simulink model "HVModAL_Fahrzeugmodell"  (R2015b)
settings: Solver=ode1  StartTime=0  StopTime=drp.driving_cycle.tstop  FixedStep=sim_params.Ts  RelTol=1e-5
PreLoadFcn:
  | % Add paths
  | addpath data
  | addpath(genpath('library'))
StartFcn:
  | Simulation.StartTime = tic;
StopFcn:
  | Simulation.DurationTime = toc(Simulation.StartTime);
undefined symbols (not defined in the file or in its folder): Batteries, BMS, BMS_Bat_, C_Nenn_DCDC1, C_Nenn_DCDC2, d2d, DC, DCDC_Converter_efficiency, DcDc_Converters, Dcl, drp, drv, elm, gen, gin, Hdc, hdc, HV, hvb, Hvb, ice, ldc, lib_dcl, lib_hdc, lib_hvb, lib_veh, Link, lossestable, mask_LUT_OCV, mask_LUT_OCV_SOC, mask_LUT_OCV_Temperature, mask_LUT_R, mask_LUT_Rs, mask_LUT_Rs_SOC, mask_LUT_Rs_Temperature, sim_params, speedvec, torquevec, tri, veh, Veh, Vehicle_Chassis
libraries: simulink x29, lib_tri_modules x7, lib_hdc_module x5, lib_gearbox x4, lib_hvb_battery_pack x3, cstblocks x3, PowerLimitBlock x2, MultiCellLibrary x2, lib_aux x1, lib_drv x1, lib_gen x1, lib_elm x1
(part 5 of 7)

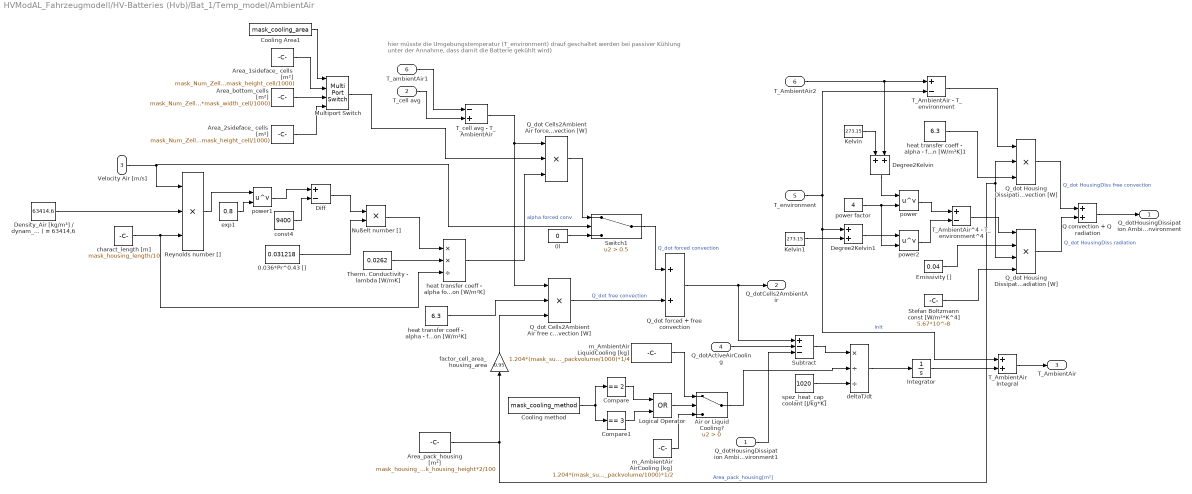
== system HVModAL_Fahrzeugmodell/HV-Batteries (Hvb)/Bat_1/Temp_model/AmbientAir ==
  note: hier müsste die Umgebungstemperatur (T_environment) drauf geschaltet werden bei passiver Kühlung
      | unter der Annahme, dass damit die Batterie gekühlt wird)
  Q_dotHousingDissipation AmbientAir2Environment1 : Inport
  T_cell avg : Inport  Port=2
  Velocity Air [m/s] : Inport  Port=3
  Q_dotActiveAirCooling : Inport  Port=4
  T_environment : Inport  Port=5
  T_AmbientAir2 : Inport  Port=6
  0.036*Pr^0.43 [] : Constant  Value=0.031218
  0l : Constant  Value=0
  Air or Liquid Cooling? : Switch  Criteria=u2 > Threshold
  Area_1sideface_ cells [m²] : Constant  Value=mask_Num_Zellen_el_ser*mask_Num_Zellen_el_par*(mask_width_cell/1000*mask_height_cell/1000)
  Area_2sideface_ cells [m²] : Constant  Value=mask_Num_Zellen_el_ser*mask_Num_Zellen_el_par*(2*mask_width_cell/1000*mask_height_cell/1000)
  Area_bottom_cells [m²] : Constant  Value=mask_Num_Zellen_el_ser*mask_Num_Zellen_el_par*(mask_thickness_cell/1000*mask_width_cell/1000)
  Area_pack_housing [m²] : Constant  Value=mask_housing_width*mask_housing_length*2/100+mask_housing_height*mask_housing_length*2/100+mask_housing_width*mask_housing_height*2/100
  Compare : simulink/Logic and Bit Operations/Compare To Constant  relop===  const=2  OutDataTypeStr=boolean
  Compare1 : simulink/Logic and Bit Operations/Compare To Constant  relop===  const=3  OutDataTypeStr=boolean
  Cooling Area1 : Constant  Value=mask_cooling_area
  Cooling method : Constant  Value=mask_cooling_method
  Degree2Kelvin : Sum
  Degree2Kelvin1 : Sum
  Density_Air [kg/m³] / dynam_visc_air @ 25°C [Pa*s] = 1,17 / (1,845*10^-5 ) = 63414,6 : Constant  Value=63414.6
  Diff : Sum  Inputs=+-
  Emissivity [] : Constant  Value=0.04
  Integrator : Integrator
  Kelvin : Constant  Value=273.15
  Kelvin1 : Constant  Value=273.15
  Logical Operator : Logic  Operator=OR  AllPortsSameDT=off  OutDataTypeStr=boolean
  Multiport Switch : MultiPortSwitch
  Nußelt number [] : Product
  Q convection + Q radiation : Sum
  Q_dot Cells2AmbientAir forced convection [W] : Product  Inputs=3
  Q_dot Cells2AmbientAir free convection [W] : Product  Inputs=3
  Q_dot Housing Dissipation free convection [W] : Product  Inputs=3
  Q_dot Housing Dissipation radiation [W] : Product  Inputs=4
  Q_dot forced + free convection : Sum
  Reynolds number [] : Product  Inputs=***
  Stefan Boltzmann const [W/m²*K^4] : Constant  Value=5.67*10^-8
  Subtract : Sum  Inputs=+--
  Switch1 : Switch  Criteria=u2 > Threshold  Threshold=0.5
  "T_AmbientAir Integral " : Sum
  T_AmbientAir - T_environment : Sum  Inputs=+-
  T_AmbientAir^4 - T_environment^4 : Sum  Inputs=+-
  T_ambientAir1 : InportShadow  Port=6
  T_cell avg - T_AmbientAir : Sum  Inputs=-+
  "Therm. Conductivity - lambda [W/mK] " : Constant  Value=0.0262
  charact_length [m] : Constant  Value=mask_housing_length/10
  const4 : Constant  Value=9400
  deltaT/dt : Product  Inputs=*//
  exp1 : Constant  Value=0.8
  factor_cell_area_housing_area : Gain  Gain=0.95
  heat transfer coeff - alpha forced convection [W/m²K] : Product  Inputs=**/
  heat transfer coeff - alpha - free convection [W/m²K] : Constant  Value=6.3
  heat transfer coeff - alpha - free convection [W/m²K]1 : Constant  Value=6.3
  m_AmbientAir AirCooling [kg] : Constant  Value=1.204*(mask_sum_packvolume/1000)*1/2
  m_AmbientAir LiquidCooling [kg] : Constant  Value=1.204*(mask_sum_packvolume/1000)*1/4
  power : Math  Operator=pow  SaturateOnIntegerOverflow=on
  power factor : Constant  Value=4
  power1 : Math  Operator=pow  SaturateOnIntegerOverflow=on
  power2 : Math  Operator=pow  SaturateOnIntegerOverflow=on
  spez_heat_cap_coolant [J/kg*K] : Constant  Value=1020
  Q_dotHousingDissipation AmbientAir2Environment : Outport
  Q_dotCells2AmbientAir : Outport  Port=2
  T_AmbientAir : Outport  Port=3
  wires:
  T_cell avg - T_AmbientAir/1 -> Q_dot Cells2AmbientAir free convection [W]/1, Q_dot Cells2AmbientAir forced convection [W]/1
  Q_dot forced + free convection/1 -> Q_dotCells2AmbientAir/1, Subtract/1
  T_cell avg/1 -> T_cell avg - T_AmbientAir/2
  Density_Air [kg/m³] / dynam_visc_air @ 25°C [Pa*s] = 1,17 / (1,845*10^-5 ) = 63414,6/1 -> Reynolds number []/2
  Reynolds number []/1 -> power1/1
  exp1/1 -> power1/2
  power1/1 -> Diff/1
  const4/1 -> Diff/2
  Diff/1 -> Nußelt number []/1
  "Therm. Conductivity - lambda [W/mK] "/1 -> heat transfer coeff - alpha forced convection [W/m²K]/2
  heat transfer coeff - alpha forced convection [W/m²K]/1 -> Q_dot Cells2AmbientAir forced convection [W]/3  "alpha forced conv"
  charact_length [m]/1 -> heat transfer coeff - alpha forced convection [W/m²K]/3, Reynolds number []/3
  Nußelt number []/1 -> heat transfer coeff - alpha forced convection [W/m²K]/1
  0.036*Pr^0.43 []/1 -> Nußelt number []/2
  Velocity Air [m/s]/1 -> Reynolds number []/1, Switch1/2
  0l/1 -> Switch1/3
  Q_dot Cells2AmbientAir forced convection [W]/1 -> Switch1/1
  Switch1/1 -> Q_dot forced + free convection/1  "Q_dot forced convection"
  Q_dot Cells2AmbientAir free convection [W]/1 -> Q_dot forced + free convection/2  "Q_dot free convection"
  heat transfer coeff - alpha - free convection [W/m²K]/1 -> Q_dot Cells2AmbientAir free convection [W]/2
  Multiport Switch/1 -> Q_dot Cells2AmbientAir forced convection [W]/2
  "T_AmbientAir Integral "/1 -> T_AmbientAir/1
  Subtract/1 -> deltaT/dt/1
  spez_heat_cap_coolant [J/kg*K]/1 -> deltaT/dt/3
  deltaT/dt/1 -> Integrator/1
  Integrator/1 -> "T_AmbientAir Integral "/2
  T_environment/1 -> T_AmbientAir - T_environment/2, Degree2Kelvin1/1, "T_AmbientAir Integral "/1  "init"
  T_AmbientAir - T_environment/1 -> Q_dot Housing Dissipation free convection [W]/1
  heat transfer coeff - alpha - free convection [W/m²K]1/1 -> Q_dot Housing Dissipation free convection [W]/3
  Area_pack_housing [m²]/1 -> Q_dot Housing Dissipation radiation [W]/3, Q_dot Housing Dissipation free convection [W]/2, factor_cell_area_housing_area/1  "Area_pack_housing[m²]"
  Q_dot Housing Dissipation free convection [W]/1 -> Q convection + Q radiation/1  "Q_dot HousingDIss free convection"
  Emissivity []/1 -> Q_dot Housing Dissipation radiation [W]/2
  Stefan Boltzmann const [W/m²*K^4]/1 -> Q_dot Housing Dissipation radiation [W]/4
  Q_dot Housing Dissipation radiation [W]/1 -> Q convection + Q radiation/2  "Q_dot HousingDiss radiation"
  Cooling method/1 -> Compare/1, Compare1/1
  Compare/1 -> Logical Operator/1
  Compare1/1 -> Logical Operator/2
  Logical Operator/1 -> Air or Liquid Cooling?/2
  Q_dotHousingDissipation AmbientAir2Environment1/1 -> Subtract/3
  power factor/1 -> power2/2, power/2
  Degree2Kelvin/1 -> power/1
  Kelvin/1 -> Degree2Kelvin/1
  T_ambientAir1/1 -> T_cell avg - T_AmbientAir/1
  T_AmbientAir2/1 -> T_AmbientAir - T_environment/1, Degree2Kelvin/2
  Q convection + Q radiation/1 -> Q_dotHousingDissipation AmbientAir2Environment/1
  Air or Liquid Cooling?/1 -> deltaT/dt/2
  m_AmbientAir AirCooling [kg]/1 -> Air or Liquid Cooling?/3
  T_AmbientAir^4 - T_environment^4/1 -> Q_dot Housing Dissipation radiation [W]/1
  power/1 -> T_AmbientAir^4 - T_environment^4/1
  Kelvin1/1 -> Degree2Kelvin1/2
  Degree2Kelvin1/1 -> power2/1
  power2/1 -> T_AmbientAir^4 - T_environment^4/2
  Q_dotActiveAirCooling/1 -> Subtract/2
  m_AmbientAir LiquidCooling [kg]/1 -> Air or Liquid Cooling?/1
  Area_bottom_cells [m²]/1 -> Multiport Switch/3
  Cooling Area1/1 -> Multiport Switch/1
  Area_1sideface_ cells [m²]/1 -> Multiport Switch/2
  Area_2sideface_ cells [m²]/1 -> Multiport Switch/4
  factor_cell_area_housing_area/1 -> Q_dot Cells2AmbientAir free convection [W]/3

== system HVModAL_Fahrzeugmodell/HV-Batteries (Hvb)/Bat_1/Temp_model/Cell ==
  Q_dot Cell2CoolingSystem+AmbientAir : Inport
  T_environment : Inport  Port=2
  Q_dot Loss Cell : Inport  Port=3
  C_Therm_Cell[J/K] : Constant  Value=1100*mask_m_cell
  Integrator : Integrator
  Q_dot Loss Cell - Q_dot Cell2CoolingSys+AmbAir : Sum  Inputs=+-
  T_cell avg Integral : Sum
  delta_T/dt : Product  Inputs=*/
  T_cell avg : Outport
  wires:
  C_Therm_Cell[J/K]/1 -> delta_T/dt/2
  delta_T/dt/1 -> Integrator/1
  Integrator/1 -> T_cell avg Integral/1
  Q_dot Loss Cell - Q_dot Cell2CoolingSys+AmbAir/1 -> delta_T/dt/1
  Q_dot Loss Cell/1 -> Q_dot Loss Cell - Q_dot Cell2CoolingSys+AmbAir/1
  T_cell avg Integral/1 -> T_cell avg/1
  Q_dot Cell2CoolingSystem+AmbientAir/1 -> Q_dot Loss Cell - Q_dot Cell2CoolingSys+AmbAir/2
  T_environment/1 -> T_cell avg Integral/2  "init"

== system HVModAL_Fahrzeugmodell/HV-Batteries (Hvb)/Bat_1/Temp_model/CoolingChannel ==
  note: 1 Elektrode Kupfer eine Alu,
      | d.h. unterschiedl. Lambdas?!
  T_environment : Inport
  T_cell avg [K] : Inport  Port=2
  Q_dot LiquidCoolingSystem : Inport  Port=3
  Q_dot PTC Heater : Inport  Port=4
  1/Thickness [1/m] : Constant  Value=1/0.006
  1/Thickness_Alu [1/m] : Constant  Value=1/0.007
  Area_1sideface_ cells [m²] : Constant  Value=mask_Num_Zellen_el_ser*mask_Num_Zellen_el_par*(mask_width_cell/1000*mask_height_cell/1000)
  Area_2sideface_ cells [m²] : Constant  Value=mask_Num_Zellen_el_ser*mask_Num_Zellen_el_par*(2*mask_width_cell/1000*mask_height_cell/1000)
  Area_bottom_cells [m²] : Constant  Value=mask_Num_Zellen_el_ser*mask_Num_Zellen_el_par*(mask_thickness_cell/1000*mask_width_cell/1000)
  Cooling Area : Constant  Value=mask_cooling_area
  Divide : Product  Inputs=*//
  Integrator : Integrator
  Multiport Switch : MultiPortSwitch
  T_ cell avg - T_Cooling Channel : Sum  Inputs=+-
  T_Cooling Channel Integral : Sum
  Temp-diff.2 : Sum  Inputs=+-
  Thermal Conductivity Alu - lambda [W/m*K] : Constant  Value=236
  Thermal Conductivity Alu - lambda [W/m*K] : Constant  Value=236
  delta_Q : Sum  Inputs=-++
  m_coolant [kg] : Constant  Value=7.28
  spez_heat_cap - c_p coolant : Constant  Value=2350
  therm conduction Cells2CoolingSystem : Product  Inputs=4
  therm_conduction Cells2Refrigerant : Product  Inputs=4
  Q_dot Cells2Refri : Outport
  Q_dot Cells2CoolingSystem : Outport  Port=2
  wires:
  Q_dot PTC Heater/1 -> delta_Q/3
  m_coolant [kg]/1 -> Divide/2
  spez_heat_cap - c_p coolant/1 -> Divide/3
  Divide/1 -> Integrator/1
  Integrator/1 -> T_Cooling Channel Integral/2
  delta_Q/1 -> Divide/1
  therm conduction Cells2CoolingSystem/1 -> Q_dot Cells2CoolingSystem/1, delta_Q/2
  1/Thickness [1/m]/1 -> therm conduction Cells2CoolingSystem/4
  T_ cell avg - T_Cooling Channel/1 -> therm conduction Cells2CoolingSystem/3
  T_Cooling Channel Integral/1 -> Temp-diff.2/1, T_ cell avg - T_Cooling Channel/2
  Thermal Conductivity Alu - lambda [W/m*K]/1 -> therm conduction Cells2CoolingSystem/2
  Q_dot LiquidCoolingSystem/1 -> delta_Q/1
  Thermal Conductivity Alu - lambda [W/m*K]/1 -> therm_conduction Cells2Refrigerant/2
  1/Thickness_Alu [1/m]/1 -> therm_conduction Cells2Refrigerant/4
  Multiport Switch/1 -> therm_conduction Cells2Refrigerant/1, therm conduction Cells2CoolingSystem/1
  Temp-diff.2/1 -> therm_conduction Cells2Refrigerant/3
  T_cell avg [K]/1 -> Temp-diff.2/2, T_ cell avg - T_Cooling Channel/1
  therm_conduction Cells2Refrigerant/1 -> Q_dot Cells2Refri/1
  T_environment/1 -> T_Cooling Channel Integral/1  "init"
  Area_bottom_cells [m²]/1 -> Multiport Switch/3
  Cooling Area/1 -> Multiport Switch/1
  Area_1sideface_ cells [m²]/1 -> Multiport Switch/2
  Area_2sideface_ cells [m²]/1 -> Multiport Switch/4

== system HVModAL_Fahrzeugmodell/HV-Batteries (Hvb)/Bat_1/Temp_model/LiquidCoolingCompressor ==
  note: 0: No cooling
      | 1: Active Aircooling
      | 2: Refrigerant Cooling
      | 3: Liquid Cooling
      | 4:Passive Aircooling
  Forced Cooled Coolant Cooling on : Inport
  Active Heating on : Inport  Port=2
  Compressor Power Factor : Inport  Port=3
  ComprCool off : Constant  Value=0
  LiquidCooling : Constant  Value=3
  Logical Op2 : Logic  AllPortsSameDT=off  OutDataTypeStr=boolean
  Null2 : Constant  Value=0
  P_max PTC Heater : Constant  Value=mask_P_max_disch*0.02
  P_max LiquidCoolingSys : Constant  Value=mask_P_max_disch*0.02
  P_max_compr [W] : Gain  Gain=mask_P_max_disch*0.02
  P_max_compr [W]1 : Gain  Gain=mask_P_max_disch*0.02
  RellOp : RelationalOperator  Operator===  OutDataTypeStr=boolean
  Switch : Switch  Criteria=u2 > Threshold  Threshold=1
  Switch3 : Switch  Criteria=u2 ~= 0  Threshold=1
  Switch4 : Switch  Criteria=u2 ~= 0  Threshold=20
  Switch5 : Switch  Criteria=u2 > Threshold  Threshold=1
  cooling system : Constant  Value=mask_cooling_method
  Q_dot LiquidCoolingSystem : Outport
  Q_dot PTC Heater : Outport  Port=2
  wires:
  P_max_compr [W]/1 -> Switch/3
  Compressor Power Factor/1 -> Switch5/2, P_max_compr [W]1/1, Switch/2, P_max_compr [W]/1
  Switch/1 -> Switch3/1
  ComprCool off/1 -> Switch3/3
  Switch4/1 -> Q_dot PTC Heater/1
  Null2/1 -> Switch4/3
  P_max PTC Heater/1 -> Switch5/1
  P_max_compr [W]1/1 -> Switch5/3
  Switch5/1 -> Switch4/1
  Switch3/1 -> Q_dot LiquidCoolingSystem/1
  Active Heating on/1 -> Switch4/2
  P_max LiquidCoolingSys/1 -> Switch/1
  cooling system/1 -> RellOp/1
  LiquidCooling/1 -> RellOp/2
  Forced Cooled Coolant Cooling on/1 -> Logical Op2/1
  RellOp/1 -> Logical Op2/2
  Logical Op2/1 -> Switch3/2

== system HVModAL_Fahrzeugmodell/HV-Batteries (Hvb)/Bat_2/BMS_Bat_/Temp Regulation ==
  note: ActiveCoolingSwitchOnTemperature
  note: @ Mitsubishi i-MiEV:
      | Active AirCooling at fastcharging with battery temperature above 30°C
      | Passive AirCooling only at battery temperature above 25°C
  note: ActiveCoolingSwitchOffTemperature
  note: ActiveHeatingSwitchOnTemperature
  note: ActiveHeatingSwitchOffTemperature
  note: 0: No cooling
      | 1: Active Aircooling
      | 2: Refrigerant Cooling
      | 3: Liquid Cooling
      | 4:Passive Aircooling
  T_max : Inport
  Fast charging on : Inport  Port=2
  Abs : Abs
  Active AirCooling : Constant
  Compare : simulink/Logic and Bit Operations/Compare To Constant  relop=>=  const=30  OutDataTypeStr=boolean
  Compare1 : simulink/Logic and Bit Operations/Compare To Constant  relop=<  const=0  OutDataTypeStr=boolean
  Cooling on : Constant  Value=4
  Gain : Gain  Gain=1/20
  Liquid Cooling : Constant  Value=3
  Logical Op1 : Logic  Operator=OR  AllPortsSameDT=off  OutDataTypeStr=boolean
  Logical Op2 : Logic  Operator=OR  AllPortsSameDT=off  OutDataTypeStr=boolean
  Logical Operator : Logic  AllPortsSameDT=off  OutDataTypeStr=boolean
  Logical Op : Logic  AllPortsSameDT=off  OutDataTypeStr=boolean
  RelOp1 : RelationalOperator  Operator===  OutDataTypeStr=boolean
  RelOp2 : RelationalOperator  Operator===  OutDataTypeStr=boolean
  Relay : Relay  OnSwitchValue=25  OffSwitchValue=20
  RellOp : RelationalOperator  Operator===  OutDataTypeStr=boolean
  Sum : Sum  Inputs=|+-
  T_desired : Constant  Value=20
  Terminator1 : Terminator
  Velocity Air [m/s] : Constant  Value=mask_v_Radial_Fan
  cooling system : Constant  Value=mask_cooling_method
  Compressor Power Factor : Outport
  Forced Air Cooling on : Outport  Port=2
  Forced Cooled Coolant Cooling on : Outport  Port=3
  Active Heating on : Outport  Port=4
  Velocity Air : Outport  Port=5
  wires:
  T_desired/1 -> Sum/1
  T_max/1 -> Compare/1, Compare1/1, Relay/1, Sum/2
  Fast charging on/1 -> Logical Operator/2
  Compare/1 -> Logical Operator/1
  Logical Operator/1 -> Terminator1/1
  Sum/1 -> Abs/1
  Abs/1 -> Gain/1
  Gain/1 -> Compressor Power Factor/1
  Cooling on/1 -> RellOp/2
  cooling system/1 -> RelOp1/1, RelOp2/1, RellOp/1
  RellOp/1 -> Logical Op2/1
  Relay/1 -> Logical Op/2
  Active AirCooling/1 -> RelOp1/2
  Liquid Cooling/1 -> RelOp2/2
  Logical Op/1 -> Forced Cooled Coolant Cooling on/1
  Compare1/1 -> Active Heating on/1
  RelOp1/1 -> Logical Op2/2, Logical Op1/1
  Velocity Air [m/s]/1 -> Velocity Air/1
  Logical Op2/1 -> Forced Air Cooling on/1
  RelOp2/1 -> Logical Op1/2
  Logical Op1/1 -> Logical Op/1

== system HVModAL_Fahrzeugmodell/HV-Batteries (Hvb)/Bat_2/Temp_model/ActiveAirCoolingCompressor ==
  note: 0: No cooling
      | 1: Active Aircooling
      | 2: Refrigerant Cooling
      | 3: Liquid Cooling
      | 4:Passive Aircooling
  ForcedAir Cooling on : Inport
  Forced Cooled Coolant Cooling on : Inport  Port=2
  Compressor Power Factor : Inport  Port=3
  Velocity Airstream : Inport  Port=4
  Active AirCooling : Constant
  Logical Op2 : Logic  AllPortsSameDT=off  OutDataTypeStr=boolean
  No convection : Constant  Value=0
  P_max LiquidCoolingSys : Constant  Value=mask_P_max_disch*0.02
  P_max_compr [W] : Gain  Gain=mask_P_max_disch*0.02
  RellOp : RelationalOperator  Operator===  OutDataTypeStr=boolean
  Switch : Switch  Criteria=u2 > Threshold  Threshold=1
  Switch1 : Switch  Criteria=u2 ~= 0  Threshold=1
  Switch3 : Switch  Criteria=u2 ~= 0  Threshold=1
  air_con_compr off : Constant  Value=0
  cooling system : Constant  Value=mask_cooling_method
  Velocity Air : Outport
  Q_dotActiveAirCooling : Outport  Port=2
  wires:
  air_con_compr off/1 -> Switch1/3
  Velocity Airstream/1 -> Switch3/1
  No convection/1 -> Switch3/3
  Switch3/1 -> Velocity Air/1
  Switch1/1 -> Q_dotActiveAirCooling/1
  ForcedAir Cooling on/1 -> Switch3/2
  P_max_compr [W]/1 -> Switch/3
  Compressor Power Factor/1 -> Switch/2, P_max_compr [W]/1
  Switch/1 -> Switch1/1
  P_max LiquidCoolingSys/1 -> Switch/1
  Forced Cooled Coolant Cooling on/1 -> Logical Op2/1
  RellOp/1 -> Logical Op2/2
  cooling system/1 -> RellOp/1
  Active AirCooling/1 -> RellOp/2
  Logical Op2/1 -> Switch1/2

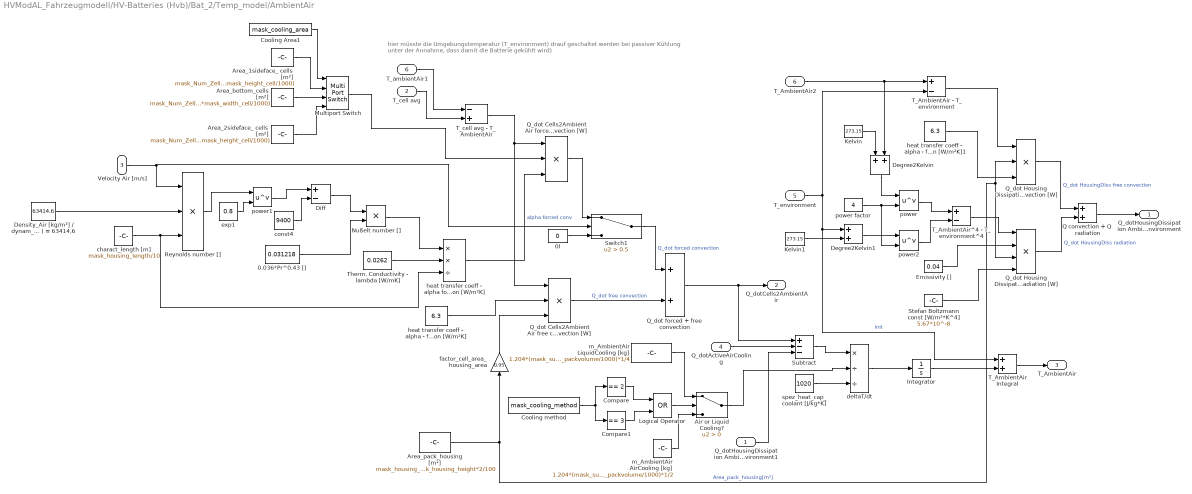
== system HVModAL_Fahrzeugmodell/HV-Batteries (Hvb)/Bat_2/Temp_model/AmbientAir ==
  note: hier müsste die Umgebungstemperatur (T_environment) drauf geschaltet werden bei passiver Kühlung
      | unter der Annahme, dass damit die Batterie gekühlt wird)
  Q_dotHousingDissipation AmbientAir2Environment1 : Inport
  T_cell avg : Inport  Port=2
  Velocity Air [m/s] : Inport  Port=3
  Q_dotActiveAirCooling : Inport  Port=4
  T_environment : Inport  Port=5
  T_AmbientAir2 : Inport  Port=6
  0.036*Pr^0.43 [] : Constant  Value=0.031218
  0l : Constant  Value=0
  Air or Liquid Cooling? : Switch  Criteria=u2 > Threshold
  Area_1sideface_ cells [m²] : Constant  Value=mask_Num_Zellen_el_ser*mask_Num_Zellen_el_par*(mask_width_cell/1000*mask_height_cell/1000)
  Area_2sideface_ cells [m²] : Constant  Value=mask_Num_Zellen_el_ser*mask_Num_Zellen_el_par*(2*mask_width_cell/1000*mask_height_cell/1000)
  Area_bottom_cells [m²] : Constant  Value=mask_Num_Zellen_el_ser*mask_Num_Zellen_el_par*(mask_thickness_cell/1000*mask_width_cell/1000)
  Area_pack_housing [m²] : Constant  Value=mask_housing_width*mask_housing_length*2/100+mask_housing_height*mask_housing_length*2/100+mask_housing_width*mask_housing_height*2/100
  Compare : simulink/Logic and Bit Operations/Compare To Constant  relop===  const=2  OutDataTypeStr=boolean
  Compare1 : simulink/Logic and Bit Operations/Compare To Constant  relop===  const=3  OutDataTypeStr=boolean
  Cooling Area1 : Constant  Value=mask_cooling_area
  Cooling method : Constant  Value=mask_cooling_method
  Degree2Kelvin : Sum
  Degree2Kelvin1 : Sum
  Density_Air [kg/m³] / dynam_visc_air @ 25°C [Pa*s] = 1,17 / (1,845*10^-5 ) = 63414,6 : Constant  Value=63414.6
  Diff : Sum  Inputs=+-
  Emissivity [] : Constant  Value=0.04
  Integrator : Integrator
  Kelvin : Constant  Value=273.15
  Kelvin1 : Constant  Value=273.15
  Logical Operator : Logic  Operator=OR  AllPortsSameDT=off  OutDataTypeStr=boolean
  Multiport Switch : MultiPortSwitch
  Nußelt number [] : Product
  Q convection + Q radiation : Sum
  Q_dot Cells2AmbientAir forced convection [W] : Product  Inputs=3
  Q_dot Cells2AmbientAir free convection [W] : Product  Inputs=3
  Q_dot Housing Dissipation free convection [W] : Product  Inputs=3
  Q_dot Housing Dissipation radiation [W] : Product  Inputs=4
  Q_dot forced + free convection : Sum
  Reynolds number [] : Product  Inputs=***
  Stefan Boltzmann const [W/m²*K^4] : Constant  Value=5.67*10^-8
  Subtract : Sum  Inputs=+--
  Switch1 : Switch  Criteria=u2 > Threshold  Threshold=0.5
  "T_AmbientAir Integral " : Sum
  T_AmbientAir - T_environment : Sum  Inputs=+-
  T_AmbientAir^4 - T_environment^4 : Sum  Inputs=+-
  T_ambientAir1 : InportShadow  Port=6
  T_cell avg - T_AmbientAir : Sum  Inputs=-+
  "Therm. Conductivity - lambda [W/mK] " : Constant  Value=0.0262
  charact_length [m] : Constant  Value=mask_housing_length/10
  const4 : Constant  Value=9400
  deltaT/dt : Product  Inputs=*//
  exp1 : Constant  Value=0.8
  factor_cell_area_housing_area : Gain  Gain=0.95
  heat transfer coeff - alpha forced convection [W/m²K] : Product  Inputs=**/
  heat transfer coeff - alpha - free convection [W/m²K] : Constant  Value=6.3
  heat transfer coeff - alpha - free convection [W/m²K]1 : Constant  Value=6.3
  m_AmbientAir AirCooling [kg] : Constant  Value=1.204*(mask_sum_packvolume/1000)*1/2
  m_AmbientAir LiquidCooling [kg] : Constant  Value=1.204*(mask_sum_packvolume/1000)*1/4
  power : Math  Operator=pow  SaturateOnIntegerOverflow=on
  power factor : Constant  Value=4
  power1 : Math  Operator=pow  SaturateOnIntegerOverflow=on
  power2 : Math  Operator=pow  SaturateOnIntegerOverflow=on
  spez_heat_cap_coolant [J/kg*K] : Constant  Value=1020
  Q_dotHousingDissipation AmbientAir2Environment : Outport
  Q_dotCells2AmbientAir : Outport  Port=2
  T_AmbientAir : Outport  Port=3
  wires:
  T_cell avg - T_AmbientAir/1 -> Q_dot Cells2AmbientAir free convection [W]/1, Q_dot Cells2AmbientAir forced convection [W]/1
  Q_dot forced + free convection/1 -> Q_dotCells2AmbientAir/1, Subtract/1
  T_cell avg/1 -> T_cell avg - T_AmbientAir/2
  Density_Air [kg/m³] / dynam_visc_air @ 25°C [Pa*s] = 1,17 / (1,845*10^-5 ) = 63414,6/1 -> Reynolds number []/2
  Reynolds number []/1 -> power1/1
  exp1/1 -> power1/2
  power1/1 -> Diff/1
  const4/1 -> Diff/2
  Diff/1 -> Nußelt number []/1
  "Therm. Conductivity - lambda [W/mK] "/1 -> heat transfer coeff - alpha forced convection [W/m²K]/2
  heat transfer coeff - alpha forced convection [W/m²K]/1 -> Q_dot Cells2AmbientAir forced convection [W]/3  "alpha forced conv"
  charact_length [m]/1 -> heat transfer coeff - alpha forced convection [W/m²K]/3, Reynolds number []/3
  Nußelt number []/1 -> heat transfer coeff - alpha forced convection [W/m²K]/1
  0.036*Pr^0.43 []/1 -> Nußelt number []/2
  Velocity Air [m/s]/1 -> Reynolds number []/1, Switch1/2
  0l/1 -> Switch1/3
  Q_dot Cells2AmbientAir forced convection [W]/1 -> Switch1/1
  Switch1/1 -> Q_dot forced + free convection/1  "Q_dot forced convection"
  Q_dot Cells2AmbientAir free convection [W]/1 -> Q_dot forced + free convection/2  "Q_dot free convection"
  heat transfer coeff - alpha - free convection [W/m²K]/1 -> Q_dot Cells2AmbientAir free convection [W]/2
  Multiport Switch/1 -> Q_dot Cells2AmbientAir forced convection [W]/2
  "T_AmbientAir Integral "/1 -> T_AmbientAir/1
  Subtract/1 -> deltaT/dt/1
  spez_heat_cap_coolant [J/kg*K]/1 -> deltaT/dt/3
  deltaT/dt/1 -> Integrator/1
  Integrator/1 -> "T_AmbientAir Integral "/2
  T_environment/1 -> T_AmbientAir - T_environment/2, Degree2Kelvin1/1, "T_AmbientAir Integral "/1  "init"
  T_AmbientAir - T_environment/1 -> Q_dot Housing Dissipation free convection [W]/1
  heat transfer coeff - alpha - free convection [W/m²K]1/1 -> Q_dot Housing Dissipation free convection [W]/3
  Area_pack_housing [m²]/1 -> Q_dot Housing Dissipation radiation [W]/3, Q_dot Housing Dissipation free convection [W]/2, factor_cell_area_housing_area/1  "Area_pack_housing[m²]"
  Q_dot Housing Dissipation free convection [W]/1 -> Q convection + Q radiation/1  "Q_dot HousingDIss free convection"
  Emissivity []/1 -> Q_dot Housing Dissipation radiation [W]/2
  Stefan Boltzmann const [W/m²*K^4]/1 -> Q_dot Housing Dissipation radiation [W]/4
  Q_dot Housing Dissipation radiation [W]/1 -> Q convection + Q radiation/2  "Q_dot HousingDiss radiation"
  Cooling method/1 -> Compare/1, Compare1/1
  Compare/1 -> Logical Operator/1
  Compare1/1 -> Logical Operator/2
  Logical Operator/1 -> Air or Liquid Cooling?/2
  Q_dotHousingDissipation AmbientAir2Environment1/1 -> Subtract/3
  power factor/1 -> power2/2, power/2
  Degree2Kelvin/1 -> power/1
  Kelvin/1 -> Degree2Kelvin/1
  T_ambientAir1/1 -> T_cell avg - T_AmbientAir/1
  T_AmbientAir2/1 -> T_AmbientAir - T_environment/1, Degree2Kelvin/2
  Q convection + Q radiation/1 -> Q_dotHousingDissipation AmbientAir2Environment/1
  Air or Liquid Cooling?/1 -> deltaT/dt/2
  m_AmbientAir AirCooling [kg]/1 -> Air or Liquid Cooling?/3
  T_AmbientAir^4 - T_environment^4/1 -> Q_dot Housing Dissipation radiation [W]/1
  power/1 -> T_AmbientAir^4 - T_environment^4/1
  Kelvin1/1 -> Degree2Kelvin1/2
  Degree2Kelvin1/1 -> power2/1
  power2/1 -> T_AmbientAir^4 - T_environment^4/2
  Q_dotActiveAirCooling/1 -> Subtract/2
  m_AmbientAir LiquidCooling [kg]/1 -> Air or Liquid Cooling?/1
  Area_bottom_cells [m²]/1 -> Multiport Switch/3
  Cooling Area1/1 -> Multiport Switch/1
  Area_1sideface_ cells [m²]/1 -> Multiport Switch/2
  Area_2sideface_ cells [m²]/1 -> Multiport Switch/4
  factor_cell_area_housing_area/1 -> Q_dot Cells2AmbientAir free convection [W]/3

== system HVModAL_Fahrzeugmodell/HV-Batteries (Hvb)/Bat_2/Temp_model/Cell ==
  Q_dot Cell2CoolingSystem+AmbientAir : Inport
  T_environment : Inport  Port=2
  Q_dot Loss Cell : Inport  Port=3
  C_Therm_Cell[J/K] : Constant  Value=1100*mask_m_cell
  Integrator : Integrator
  Q_dot Loss Cell - Q_dot Cell2CoolingSys+AmbAir : Sum  Inputs=+-
  T_cell avg Integral : Sum
  delta_T/dt : Product  Inputs=*/
  T_cell avg : Outport
  wires:
  C_Therm_Cell[J/K]/1 -> delta_T/dt/2
  delta_T/dt/1 -> Integrator/1
  Integrator/1 -> T_cell avg Integral/1
  Q_dot Loss Cell - Q_dot Cell2CoolingSys+AmbAir/1 -> delta_T/dt/1
  Q_dot Loss Cell/1 -> Q_dot Loss Cell - Q_dot Cell2CoolingSys+AmbAir/1
  T_cell avg Integral/1 -> T_cell avg/1
  Q_dot Cell2CoolingSystem+AmbientAir/1 -> Q_dot Loss Cell - Q_dot Cell2CoolingSys+AmbAir/2
  T_environment/1 -> T_cell avg Integral/2  "init"

== system HVModAL_Fahrzeugmodell/HV-Batteries (Hvb)/Bat_2/Temp_model/CoolingChannel ==
  note: 1 Elektrode Kupfer eine Alu,
      | d.h. unterschiedl. Lambdas?!
  T_environment : Inport
  T_cell avg [K] : Inport  Port=2
  Q_dot LiquidCoolingSystem : Inport  Port=3
  Q_dot PTC Heater : Inport  Port=4
  1/Thickness [1/m] : Constant  Value=1/0.006
  1/Thickness_Alu [1/m] : Constant  Value=1/0.007
  Area_1sideface_ cells [m²] : Constant  Value=mask_Num_Zellen_el_ser*mask_Num_Zellen_el_par*(mask_width_cell/1000*mask_height_cell/1000)
  Area_2sideface_ cells [m²] : Constant  Value=mask_Num_Zellen_el_ser*mask_Num_Zellen_el_par*(2*mask_width_cell/1000*mask_height_cell/1000)
  Area_bottom_cells [m²] : Constant  Value=mask_Num_Zellen_el_ser*mask_Num_Zellen_el_par*(mask_thickness_cell/1000*mask_width_cell/1000)
  Cooling Area : Constant  Value=mask_cooling_area
  Divide : Product  Inputs=*//
  Integrator : Integrator
  Multiport Switch : MultiPortSwitch
  T_ cell avg - T_Cooling Channel : Sum  Inputs=+-
  T_Cooling Channel Integral : Sum
  Temp-diff.2 : Sum  Inputs=+-
  Thermal Conductivity Alu - lambda [W/m*K] : Constant  Value=236
  Thermal Conductivity Alu - lambda [W/m*K] : Constant  Value=236
  delta_Q : Sum  Inputs=-++
  m_coolant [kg] : Constant  Value=7.28
  spez_heat_cap - c_p coolant : Constant  Value=2350
  therm conduction Cells2CoolingSystem : Product  Inputs=4
  therm_conduction Cells2Refrigerant : Product  Inputs=4
  Q_dot Cells2Refri : Outport
  Q_dot Cells2CoolingSystem : Outport  Port=2
  wires:
  Q_dot PTC Heater/1 -> delta_Q/3
  m_coolant [kg]/1 -> Divide/2
  spez_heat_cap - c_p coolant/1 -> Divide/3
  Divide/1 -> Integrator/1
  Integrator/1 -> T_Cooling Channel Integral/2
  delta_Q/1 -> Divide/1
  therm conduction Cells2CoolingSystem/1 -> Q_dot Cells2CoolingSystem/1, delta_Q/2
  1/Thickness [1/m]/1 -> therm conduction Cells2CoolingSystem/4
  T_ cell avg - T_Cooling Channel/1 -> therm conduction Cells2CoolingSystem/3
  T_Cooling Channel Integral/1 -> Temp-diff.2/1, T_ cell avg - T_Cooling Channel/2
  Thermal Conductivity Alu - lambda [W/m*K]/1 -> therm conduction Cells2CoolingSystem/2
  Q_dot LiquidCoolingSystem/1 -> delta_Q/1
  Thermal Conductivity Alu - lambda [W/m*K]/1 -> therm_conduction Cells2Refrigerant/2
  1/Thickness_Alu [1/m]/1 -> therm_conduction Cells2Refrigerant/4
  Multiport Switch/1 -> therm_conduction Cells2Refrigerant/1, therm conduction Cells2CoolingSystem/1
  Temp-diff.2/1 -> therm_conduction Cells2Refrigerant/3
  T_cell avg [K]/1 -> Temp-diff.2/2, T_ cell avg - T_Cooling Channel/1
  therm_conduction Cells2Refrigerant/1 -> Q_dot Cells2Refri/1
  T_environment/1 -> T_Cooling Channel Integral/1  "init"
  Area_bottom_cells [m²]/1 -> Multiport Switch/3
  Cooling Area/1 -> Multiport Switch/1
  Area_1sideface_ cells [m²]/1 -> Multiport Switch/2
  Area_2sideface_ cells [m²]/1 -> Multiport Switch/4

== system HVModAL_Fahrzeugmodell/HV-Batteries (Hvb)/Bat_2/Temp_model/LiquidCoolingCompressor ==
  note: 0: No cooling
      | 1: Active Aircooling
      | 2: Refrigerant Cooling
      | 3: Liquid Cooling
      | 4:Passive Aircooling
  Forced Cooled Coolant Cooling on : Inport
  Active Heating on : Inport  Port=2
  Compressor Power Factor : Inport  Port=3
  ComprCool off : Constant  Value=0
  LiquidCooling : Constant  Value=3
  Logical Op2 : Logic  AllPortsSameDT=off  OutDataTypeStr=boolean
  Null2 : Constant  Value=0
  P_max PTC Heater : Constant  Value=mask_P_max_disch*0.02
  P_max LiquidCoolingSys : Constant  Value=mask_P_max_disch*0.02
  P_max_compr [W] : Gain  Gain=mask_P_max_disch*0.02
  P_max_compr [W]1 : Gain  Gain=mask_P_max_disch*0.02
  RellOp : RelationalOperator  Operator===  OutDataTypeStr=boolean
  Switch : Switch  Criteria=u2 > Threshold  Threshold=1
  Switch3 : Switch  Criteria=u2 ~= 0  Threshold=1
  Switch4 : Switch  Criteria=u2 ~= 0  Threshold=20
  Switch5 : Switch  Criteria=u2 > Threshold  Threshold=1
  cooling system : Constant  Value=mask_cooling_method
  Q_dot LiquidCoolingSystem : Outport
  Q_dot PTC Heater : Outport  Port=2
  wires:
  P_max_compr [W]/1 -> Switch/3
  Compressor Power Factor/1 -> Switch5/2, P_max_compr [W]1/1, Switch/2, P_max_compr [W]/1
  Switch/1 -> Switch3/1
  ComprCool off/1 -> Switch3/3
  Switch4/1 -> Q_dot PTC Heater/1
  Null2/1 -> Switch4/3
  P_max PTC Heater/1 -> Switch5/1
  P_max_compr [W]1/1 -> Switch5/3
  Switch5/1 -> Switch4/1
  Switch3/1 -> Q_dot LiquidCoolingSystem/1
  Active Heating on/1 -> Switch4/2
  P_max LiquidCoolingSys/1 -> Switch/1
  cooling system/1 -> RellOp/1
  LiquidCooling/1 -> RellOp/2
  Forced Cooled Coolant Cooling on/1 -> Logical Op2/1
  RellOp/1 -> Logical Op2/2
  Logical Op2/1 -> Switch3/2

== system HVModAL_Fahrzeugmodell/Traction Inverters (Tri)/Tri1/Control Unit/Thermal Control ==
  Tri_at_Junction : Inport
  at_Ambient : Inport  Port=2
  Pmax_cold : Constant  Value=TRIname.Pmax
  Pmax_warm : Constant  Value=TRIname.Pmax*0.75
  Switch : Switch  Criteria=u2 > Threshold  Threshold=140
  Terminator3 : Terminator
  Pmax : Outport
  wires:
  Tri_at_Junction/1 -> Switch/2
  Pmax_cold/1 -> Switch/3
  Switch/1 -> Pmax/1
  Pmax_warm/1 -> Switch/1
  at_Ambient/1 -> Terminator3/1

== system HVModAL_Fahrzeugmodell/Traction Inverters (Tri)/Tri1/Thermal Model/Conventional thermal model ==
  P_loss_vec : Inport
  T_amb : Inport  Port=2
  Enable : EnablePort
  Conventional thermal model : Subsystem
  Conventional thermal model1 : lib_tri_modules/Tri/Thermal Model/Conventional thermal model/Conventional thermal model
  Conventional thermal model2 : lib_tri_modules/Tri/Thermal Model/Conventional thermal model/Conventional thermal model
  Demux : Demux  Outputs=12
  Mux : Mux
  Mux1 : Mux
  Mux2 : Mux
  Mux3 : Mux  Inputs=3
  T_junction : Outport
  wires:
  P_loss_vec/1 -> Demux/1
  Conventional thermal model/1(Temperature) -> Mux3/1
  T_amb/1 -> Conventional thermal model2/2, Conventional thermal model1/2, Conventional thermal model/2(T_amb)
  Demux/1 -> Mux/1
  Demux/2 -> Mux/2
  Demux/3 -> Mux/3
  Demux/4 -> Mux/4
  Demux/5 -> Mux1/1
  Demux/6 -> Mux1/2
  Demux/7 -> Mux1/3
  Demux/8 -> Mux1/4
  Demux/9 -> Mux2/1
  Demux/10 -> Mux2/2
  Demux/11 -> Mux2/3
  Demux/12 -> Mux2/4
  Mux/1 -> Conventional thermal model/1(P losses)
  Mux3/1 -> T_junction/1
  Mux2/1 -> Conventional thermal model2/1
  Mux1/1 -> Conventional thermal model1/1
  Conventional thermal model1/1 -> Mux3/2
  Conventional thermal model2/1 -> Mux3/3

== system HVModAL_Fahrzeugmodell/Traction Inverters (Tri)/Tri1/Thermal Model/Foster Model ==
  P_loss_vec : Inport
  T_amb : Inport  Port=2
  Enable : EnablePort
  Add : Sum
  Demux : Demux  Outputs=3
  Leg1 : Subsystem
  Leg2 : lib_tri_modules/Tri/Thermal Model/Foster Model/Leg1
  Leg3 : lib_tri_modules/Tri/Thermal Model/Foster Model/Leg1
  Mux : Mux  Inputs=3
  T_junction : Outport
  wires:
  Demux/2 -> Leg2/1
  Add/1 -> T_junction/1
  T_amb/1 -> Add/2
  P_loss_vec/1 -> Demux/1
  Demux/3 -> Leg3/1
  Demux/1 -> Leg1/1(In1)
  Mux/1 -> Add/1
  Leg3/1 -> Mux/3
  Leg2/1 -> Mux/2
  Leg1/1(Leg1TempVec) -> Mux/1

== system HVModAL_Fahrzeugmodell/Traction Inverters (Tri)/Tri1/Thermal Model/Thermal Junction Model ==
  P_loss_vec : Inport
  T_amb : Inport  Port=2
  Enable : EnablePort
  Demux1 : Demux
  Demux2 : Demux  Outputs=[1 1 1 1 1 1 1 1 1 1 1 1]
  Demux3 : Demux
  Demux4 : Demux
  Leg 1 : cstblocks/LTI System  sys=d2d(TRIname.ThermalModel.junction.PlantJunction, sim_params.Ts)  IC=[]
  Leg 2 : cstblocks/LTI System  sys=d2d(TRIname.ThermalModel.junction.PlantJunction, sim_params.Ts)  IC=[]
  Leg 3 : cstblocks/LTI System  sys=d2d(TRIname.ThermalModel.junction.PlantJunction, sim_params.Ts)  IC=[]
  Mux : Mux  Inputs=[1 1 1 1]
  Mux1 : Mux  Inputs=[1 1 1 1 1 1 1 1 1 1 1 1]
  Mux2 : Mux  Inputs=[1 1 1 1]
  Mux3 : Mux  Inputs=[1 1 1 1]
  Sum2 : Sum  Inputs=|++  SaturateOnIntegerOverflow=on
  T_junction : Outport
  wires:
  Demux2/1 -> Mux/1  "Switch_up"
  Demux2/3 -> Mux/3  "Switch_down"
  Demux1/1 -> Mux1/1
  Demux1/2 -> Mux1/2
  Demux1/3 -> Mux1/3
  Demux1/4 -> Mux1/4
  Demux3/1 -> Mux1/5
  Demux3/2 -> Mux1/6
  Demux3/3 -> Mux1/7
  Demux3/4 -> Mux1/8
  Demux4/1 -> Mux1/9
  Demux4/2 -> Mux1/10
  Demux4/3 -> Mux1/11
  Demux4/4 -> Mux1/12
  Demux2/5 -> Mux2/1
  Demux2/6 -> Mux2/2
  Demux2/7 -> Mux2/3
  Demux2/8 -> Mux2/4
  Demux2/9 -> Mux3/1
  Demux2/10 -> Mux3/2
  Demux2/11 -> Mux3/3
  Demux2/12 -> Mux3/4
  Leg 1/1 -> Demux1/1
  Mux1/1 -> Sum2/1
  T_amb/1 -> Sum2/2
  Sum2/1 -> T_junction/1
  P_loss_vec/1 -> Demux2/1
  Mux2/1 -> Leg 2/1
  Mux3/1 -> Leg 3/1
  Leg 3/1 -> Demux4/1
  Demux2/2 -> Mux/2  "Diode_up"
  Demux2/4 -> Mux/4  "Diode_down"
  Mux/1 -> Leg 1/1
  Leg 2/1 -> Demux3/1

== system HVModAL_Fahrzeugmodell/Traction Inverters (Tri)/Tri1/Thermal Model old/Thermal Junction Model ==
  P_loss_vec : Inport
  T_amb : Inport  Port=2
  Constant : Constant  Value=3
  Constant1 : Constant  Value=0
  Demux1 : Demux
  Demux2 : Demux  Outputs=[1 1 1 1 1 1 1 1 1 1 1 1]
  Demux3 : Demux
  Demux4 : Demux
  Leg 1 : Subsystem
      mask help: Simulink:masks:GenSFuncDesc_MD
      mask Help: eval('feval(''rtwprivate'',''rtwhelpview'',''rtw_sfcn_block'')');
  Leg 2 : Subsystem
      mask help: Simulink:masks:GenSFuncDesc_MD
      mask Help: eval('feval(''rtwprivate'',''rtwhelpview'',''rtw_sfcn_block'')');
  Leg 3 : Subsystem
      mask help: Simulink:masks:GenSFuncDesc_MD
      mask Help: eval('feval(''rtwprivate'',''rtwhelpview'',''rtw_sfcn_block'')');
  Mux : Mux  Inputs=[1 1 1 1]
  Mux1 : Mux  Inputs=[1 1 1 1 1 1 1 1 1 1 1 1]
  Mux2 : Mux  Inputs=[1 1 1 1]
  Mux3 : Mux  Inputs=[1 1 1 1]
  Product : Product
  Scope : Scope
  Sum : Sum  Inputs=|++
  Sum1 : Sum  Inputs=|++  SaturateOnIntegerOverflow=on
  Sum2 : Sum  Inputs=|++  SaturateOnIntegerOverflow=on
  T_junction : Outport
  wires:
  Demux2/1 -> Mux/1  "Switch_up"
  Demux2/3 -> Mux/3  "Switch_down"
  Demux1/1 -> Mux1/1
  Demux1/2 -> Mux1/2
  Demux1/3 -> Mux1/3
  Demux1/4 -> Mux1/4
  Demux3/1 -> Mux1/5
  Demux3/2 -> Mux1/6
  Demux3/3 -> Mux1/7
  Demux3/4 -> Mux1/8
  Demux4/1 -> Mux1/9
  Demux4/2 -> Mux1/10
  Demux4/3 -> Mux1/11
  Demux4/4 -> Mux1/12
  Demux2/5 -> Mux2/1
  Demux2/6 -> Mux2/2
  Demux2/7 -> Mux2/3
  Demux2/8 -> Mux2/4
  Demux2/9 -> Mux3/1
  Demux2/10 -> Mux3/2
  Demux2/11 -> Mux3/3
  Demux2/12 -> Mux3/4
  Leg 1/1(Out1) -> Sum1/1, Demux1/1
  Mux1/1 -> Sum2/1
  T_amb/1 -> Sum2/2, Sum1/2
  Sum2/1 -> T_junction/1
  Constant/1 -> Product/2
  Product/1 -> Sum/1
  Sum/1 -> Demux2/1
  Constant1/1 -> Sum/2
  P_loss_vec/1 -> Product/1
  Mux2/1 -> Leg 2/1(In1)
  Mux3/1 -> Leg 3/1(In1)
  Leg 2/1(Out1) -> Demux3/1
  Leg 3/1(Out1) -> Demux4/1
  Demux2/2 -> Mux/2  "Diode_up"
  Demux2/4 -> Mux/4  "Diode_down"
  Mux/1 -> Leg 1/1(In1)
  Sum1/1 -> Scope/1

== system HVModAL_Fahrzeugmodell/Vehicle_Chassis (Veh)/Wheel Model/ /If Action Subsystem ==
  Action Port : ActionPort  ActionType=then
  Constant : Constant  Value=false
  Data Store Write : DataStoreWrite  DataStoreName=Slip
  wires:
  Constant/1 -> Data Store Write/1

== system HVModAL_Fahrzeugmodell/Energy Manager (Emg)/Battery Control/Driving_Mode/Range_extender 1/mapping1 ==
  P_max_ch_W_Bat1 : Inport
  P_max_Disch_W_Bat1 : Inport  Port=2
  Gain : Gain  Gain=-1
  P_LB_Bat1 : Outport
  P_UB_Bat1 : Outport  Port=2
  wires:
  Gain/1 -> P_LB_Bat1/1
  P_max_ch_W_Bat1/1 -> Gain/1
  P_max_Disch_W_Bat1/1 -> P_UB_Bat1/1

== system HVModAL_Fahrzeugmodell/Energy Manager (Emg)/Battery Control/Driving_Mode/Range_extender 1/power_distribution_new ==
  note: 5/3
  note: -2/3
  note: entladen 3000
  note: rekuperieren: -10000
  note: -0,5
  note: 1,5
  note: entladen: 10000
  P_Load_W : Inport
  P_UB_Bat1 : Inport  Port=2
  P_LB_Bat1 : Inport  Port=3
  Use_range_extender : Inport  Port=4
  P_discharge_W : Inport  Port=5
  Chart : Stateflow chart  TreatAsAtomicUnit=on
      settings: PermitHierarchicalResolution=ParametersOnly
  Chart2 : Stateflow chart  TreatAsAtomicUnit=on
      settings: PermitHierarchicalResolution=ParametersOnly
  Constant2 : Constant  Value=0
  Divide : Product  Inputs=*/
  Divide1 : Product  Inputs=*/
  Mux : Mux  Inputs=3
  P_Bat2 : Scope
  P_UB_Bat1#1 : Scope  NumInputPorts=2
  Product : Product
  Product1 : Product
  Subsystem : Subsystem
  Subtract : Sum  Inputs=+-
  abs2perc : Gain  Gain=100
  abs2perc1 : Gain  Gain=100
  abs2perc2 : Gain  Gain=100
  compare : Scope  NumInputPorts=2
  vector_PowerDistribution : Outport
  wires:
  Mux/1 -> vector_PowerDistribution/1
  abs2perc2/1 -> Mux/3  "PowerShare_Bat3"
  abs2perc/1 -> Mux/1  "PowerShare_Bat1"
  abs2perc1/1 -> Mux/2  "PowerShare_Bat2"
  Constant2/1 -> abs2perc2/1
  P_LB_Bat1/1 -> Chart/3(P_LB_Bat1)
  P_UB_Bat1/1 -> Chart/2(P_UB_Bat1)
  Subtract/1 -> Chart/1(p_Bat1_o)
  Chart/1(P_Bat1) -> Divide1/1
  Use_range_extender/1 -> Product/2
  Divide1/1 -> compare/1, abs2perc/1
  P_discharge_W/1 -> Product/1
  Product1/1 -> P_Bat2/1
  Subsystem/1(P_Bat2) -> Subtract/2, Divide/1
  Product/1 -> Subsystem/2(P_Bat2_discharge_max)
  Divide/1 -> abs2perc1/1, Product1/1, compare/2
  P_Load_W/1 -> Product1/2, Subtract/1, Divide1/2, Divide/2, P_UB_Bat1#1/1, P_UB_Bat1#1/2, Subsystem/1(P_load)

== system HVModAL_Fahrzeugmodell/Energy Manager (Emg)/Battery Control/Driving_Mode/Range_extender 1/power_distribution_old ==
  P_Load_W : Inport
  P2_discharge_W : Inport  Port=2
  Use_Range_extender : Inport  Port=3
  P_UB_Bat1 : Inport  Port=4
  P_LB_Bat1 : Inport  Port=5
  Chart : Stateflow chart  TreatAsAtomicUnit=on
      settings: PermitHierarchicalResolution=ParametersOnly
  Constant2 : Constant  Value=0
  Divide : Product  Inputs=*/
  Divide1 : Product  Inputs=*/
  Mux : Mux  Inputs=3
  P_Bat1 : Scope
  P_LB_Bat1# : Scope
  P_UB_Bat1# : Scope
  Product : Product
  Subtract : Sum  Inputs=+-
  abs2perc : Gain  Gain=100
  abs2perc1 : Gain  Gain=100
  abs2perc2 : Gain  Gain=100
  vector_PowerDistribution : Outport
  wires:
  Mux/1 -> vector_PowerDistribution/1
  abs2perc2/1 -> Mux/3  "PowerShare_Bat3"
  abs2perc/1 -> Mux/1  "PowerShare_Bat1"
  abs2perc1/1 -> Mux/2  "PowerShare_Bat2"
  Constant2/1 -> abs2perc2/1
  P2_discharge_W/1 -> Product/1
  Divide1/1 -> abs2perc/1
  Product/1 -> Subtract/2, Divide/1
  Use_Range_extender/1 -> Product/2
  Divide/1 -> abs2perc1/1
  P_LB_Bat1/1 -> P_LB_Bat1#/1, Chart/3(P_LB_Bat1)
  P_UB_Bat1/1 -> P_UB_Bat1#/1, Chart/2(P_UB_Bat1)
  Subtract/1 -> Chart/1(p_Bat1_o)
  Chart/1(P_Bat1) -> Divide1/1, P_Bat1/1
  P_Load_W/1 -> Divide/2, Divide1/2, Subtract/1

== system HVModAL_Fahrzeugmodell/Energy Manager (Emg)/Battery Control/Driving_Mode/Range_extender 2/dynamic ==
  note: dynamic mode:
  note: Range extender 5kw
  P_max_Disch_W_Bat2 : Inport
  P_currentPower_W_Bat1 : Inport  Port=2
  P_currentPower_W_Bat2 : Inport  Port=3
  P_currentPower_W_Bat3 : Inport  Port=4
  P_max_ch_W_Bat1 : Inport  Port=5
  P_max_Disch_W_Bat1 : Inport  Port=6
  SOC_perc_01 : Inport  Port=7
  SOC_perc_02 : Inport  Port=8
  cell number : Inport  Port=9
  bat1_kwh : Inport  Port=10
  driving_range : Inport  Port=11
  city_1_or_highway_0 : Inport  Port=12
  I_bat2_A : Inport  Port=13
  P_currentPower_Inv_W : Inport  Port=14
  P_currentPower_Aux_W : Inport  Port=15
  T_Cell_avg : Inport  Port=16
  Action Port : ActionPort  ActionType=default
  Scope : Scope
  Scope1 : Scope
  Scope2 : Scope
  "power estimination " : Subsystem
  power_distribution_new : Subsystem
  "soc estimination " : Subsystem
  vector_PowerDistribution : Outport
  wires:
  P_max_ch_W_Bat1/1 -> "power estimination "/5(P_max_ch_W_Bat1)
  driving_range/1 -> "soc estimination "/1(driving range)
  SOC_perc_02/1 -> "soc estimination "/3(soc_perc_02)
  "soc estimination "/1("Turn_on_rex ") -> [Turn_on_range_extender]
  P_currentPower_W_Bat1/1 -> "power estimination "/2(P_currentPower_W_Bat1)
  P_currentPower_W_Bat2/1 -> "power estimination "/3(P_currentPower_W_Bat2)
  P_currentPower_W_Bat3/1 -> "power estimination "/4(P_currentPower_W_Bat3)
  P_max_Disch_W_Bat2/1 -> "power estimination "/1(P_max_Disch_W_Bat2)
  "power estimination "/2(P_Load_W) -> Scope1/1, [P_Load_W]
  "power estimination "/3(P_LB_Bat1) -> [P_LB_Bat1]
  "power estimination "/4(P_UB_Bat1) -> [P_UB_Bat1]
  "power estimination "/1(p_bat2) -> [p_bat2]
  P_max_Disch_W_Bat1/1 -> "power estimination "/6(P_max_Disch_W_Bat1)
  [p_bat2] -> power_distribution_new/5(P_bat2_W)
  [P_Load_W] -> Scope2/1, power_distribution_new/1(P_Load_W)
  [P_UB_Bat1] -> power_distribution_new/2(P_UB_Bat1)
  [P_LB_Bat1] -> power_distribution_new/3(P_LB_Bat1)
  power_distribution_new/1(vector_PowerDistribution) -> vector_PowerDistribution/1
  [Turn_on_range_extender] -> power_distribution_new/4(Turn_on_range_extender)
  SOC_perc_01/1 -> "soc estimination "/2(soc_perc_01)
  bat1_kwh/1 -> "soc estimination "/4(bat1)
  cell number/1 -> "soc estimination "/5(cell number)
  city_1_or_highway_0/1 -> "soc estimination "/6(city or highway), power_distribution_new/6(city_1_or_highway_0)
  I_bat2_A/1 -> Scope/1
  P_currentPower_Inv_W/1 -> "power estimination "/8(P_currentPower_Inv_W)
  P_currentPower_Aux_W/1 -> "power estimination "/9(P_currentPower_Aux_W)
  "soc estimination "/2(I_rex 1) -> [I_rex]
  [I_rex] -> "power estimination "/7("I_rex ")
  T_Cell_avg/1 -> power_distribution_new/7(T_Cell_avg)

== system HVModAL_Fahrzeugmodell/Energy Manager (Emg)/Battery Control/Driving_Mode/Range_extender 2/start_from_30% 1 ==
  note: Range extender 5kw
  P_currentPower_W_Bat1 : Inport
  P_currentPower_W_Bat2 : Inport  Port=2
  P_currentPower_W_Bat3 : Inport  Port=3
  P_max_ch_W_Bat1 : Inport  Port=4
  P_max_Disch_W_Bat1 : Inport  Port=5
  SOC_perc_01 : Inport  Port=6
  SOC_perc_02 : Inport  Port=7
  P_max_Disch_W_Bat2 : Inport  Port=8
  bat_1_Wh : Inport  Port=9
  driving_range : Inport  Port=10
  Veh_v_actual : Inport  Port=11
  P_currentPower_Inv_W : Inport  Port=12
  P_currentPower_Aux_W : Inport  Port=13
  T_Cell_avg : Inport  Port=14
  Action Port : ActionPort  ActionType=case
  Scope : Scope
  Scope1 : Scope
  "power estimination " : Subsystem
  power_distribution_new : Subsystem
  "soc estimination " : Subsystem
  vector_PowerDistribution : Outport
  tag scope: I_rex_global3=global
  wires:
  P_max_ch_W_Bat1/1 -> "power estimination "/4(P_max_ch_W_Bat1)
  SOC_perc_02/1 -> "soc estimination "/2(soc_perc_02)
  "soc estimination "/1("Turn_on_rex ") -> Scope/1, [Turn_on_range_extender]
  P_currentPower_W_Bat1/1 -> "power estimination "/1(P_currentPower_W_Bat1)
  P_currentPower_W_Bat2/1 -> "power estimination "/2(P_currentPower_W_Bat2)
  P_currentPower_W_Bat3/1 -> "power estimination "/3(P_currentPower_W_Bat3)
  "power estimination "/1(P_Load_W) -> [P_Load_W]
  "power estimination "/2(P_LB_Bat1) -> [P_LB_Bat1]
  "power estimination "/3(P_UB_Bat1) -> [P_UB_Bat1]
  P_max_Disch_W_Bat1/1 -> "power estimination "/5(P_max_Disch_W_Bat1)
  [P_Load_W] -> power_distribution_new/1(P_Load_W)
  [P_UB_Bat1] -> power_distribution_new/2(P_UB_Bat1)
  [P_LB_Bat1] -> power_distribution_new/3(P_LB_Bat1)
  power_distribution_new/1(vector_PowerDistribution) -> vector_PowerDistribution/1
  [Turn_on_range_extender] -> power_distribution_new/4(Turn_on_range_extender)
  SOC_perc_01/1 -> "soc estimination "/1(soc_perc_01)
  [p_bat2] -> Scope1/1, power_distribution_new/5(P_discharge_W)
  P_max_Disch_W_Bat2/1 -> "power estimination "/6(P_max_Disch_W_Bat2)
  "power estimination "/4(p_bat2) -> [p_bat2]
  "soc estimination "/2(I_rex 1) -> [I_rex_global3]
  driving_range/1 -> "soc estimination "/4(driving range)
  bat_1_Wh/1 -> "soc estimination "/3(bat1)
  Veh_v_actual/1 -> "soc estimination "/5(Veh_v_actual)
  P_currentPower_Inv_W/1 -> "power estimination "/8(P_currentPower_Inv_W)
  P_currentPower_Aux_W/1 -> "power estimination "/9(P_currentPower_Aux_W)
  [I_rex_global3] -> "power estimination "/7("I_rex ")
  T_Cell_avg/1 -> power_distribution_new/6(T_Cell_avg)

== system HVModAL_Fahrzeugmodell/Energy Manager (Emg)/Battery Control/Driving_Mode/Range_extender 2/start_from_begining  ==
  note: Range extender 5kw
  P_max_ch_W_Bat1 : Inport
  P_max_Disch_W_Bat1 : Inport  Port=2
  SOC_perc_01 : Inport  Port=3
  SOC_perc_02 : Inport  Port=4
  P_max_Disch_W_Bat2 : Inport  Port=5
  bat_1_Wh : Inport  Port=6
  driving range : Inport  Port=7
  " city_1_or_highway_0" : Inport  Port=8
  P_currentPower_Aux_W : Inport  Port=9
  P_currentPower_Inv_W : Inport  Port=10
  T_Cell_avg : Inport  Port=11
  Action Port : ActionPort  ActionType=case
  Scope : Scope
  Scope1 : Scope
  Scope3 : Scope
  "power estimination " : Subsystem
  power_distribution_new : Subsystem
  "soc estimination " : Subsystem
  vector_PowerDistribution : Outport
  tag scope: I_REX_global2=global
  wires:
  P_max_ch_W_Bat1/1 -> "power estimination "/1(P_max_ch_W_Bat1)
  SOC_perc_02/1 -> "soc estimination "/2(soc_perc_02)
  "soc estimination "/1("Turn_on_rex ") -> Scope/1, [Turn_on_range_extender]
  "power estimination "/4(P_Load_W) -> [P_Load_W]
  "power estimination "/1(P_LB_Bat1) -> [P_LB_Bat1]
  "power estimination "/2(P_UB_Bat1) -> [P_UB_Bat1]
  P_max_Disch_W_Bat1/1 -> "power estimination "/2(P_max_Disch_W_Bat1)
  [P_Load_W] -> power_distribution_new/1(P_Load_W)
  [P_UB_Bat1] -> power_distribution_new/2(P_UB_Bat1)
  [P_LB_Bat1] -> power_distribution_new/3(P_LB_Bat1)
  power_distribution_new/1(vector_PowerDistribution) -> vector_PowerDistribution/1
  [Turn_on_range_extender] -> power_distribution_new/4(Turn_on_range_extender)
  SOC_perc_01/1 -> "soc estimination "/1(soc_perc_01)
  [p_bat2] -> power_distribution_new/5(P_discharge_W), Scope1/1
  P_max_Disch_W_Bat2/1 -> "power estimination "/3(P_max_Disch_W_Bat2)
  "power estimination "/3(p_bat2) -> [p_bat2]
  "soc estimination "/2(I_rex 1) -> [I_REX_global2]
  bat_1_Wh/1 -> "soc estimination "/3(bat1)
  driving range/1 -> "soc estimination "/4(driving range)
  " city_1_or_highway_0"/1 -> "soc estimination "/5(city_1_or_highway_0), power_distribution_new/6(city_1_or_highway_0)
  [I_REX_global2] -> "power estimination "/4("I_rex ")
  P_currentPower_Aux_W/1 -> "power estimination "/6(P_currentPower_Aux_W)
  T_Cell_avg/1 -> power_distribution_new/7(T_Cell_avg)
